simulink model "uncontrolled_test"  (R2020b)
settings: Solver=VariableStepAuto  StartTime=0.0  StopTime=5000  RelTol=1e-3
values from neighbouring files (symbols this model uses):
  spacecraft = struct()    [setup.m]
undefined symbols (not defined in the file or in its folder): constants
libraries: library x5, vrlib x3
settings Model: Creator=loren  LastModifiedBy=loren

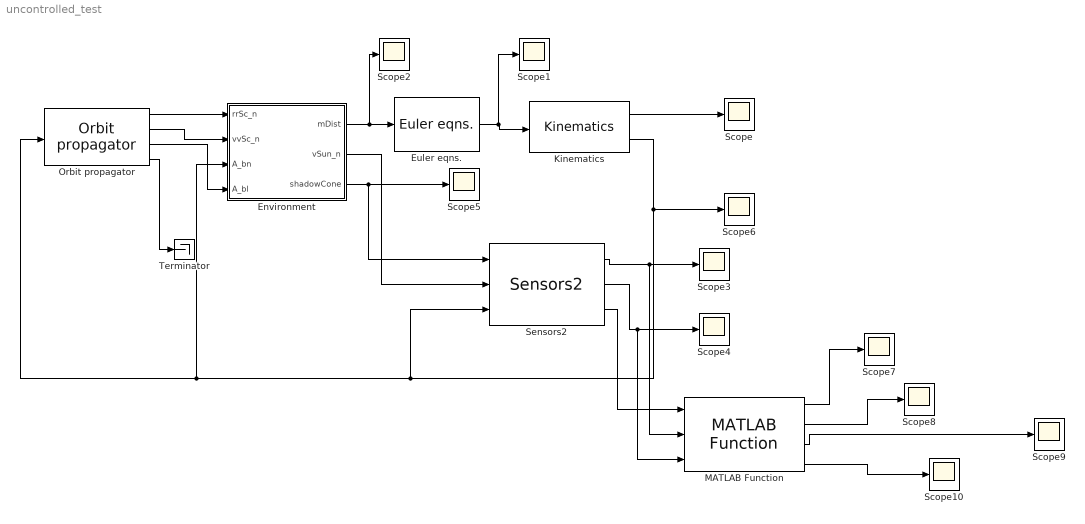
== system uncontrolled_test ==
  Environment : Subsystem  AncestorBlock=library/Environment
  Euler eqns. : library/Euler eqns.  SystemSampleTime=-1  VariantActivationTime=update diagram  Latency=0  AutoFrameSizeCalculation=off
  Kinematics : library/Kinematics  SystemSampleTime=-1  VariantActivationTime=update diagram  Latency=0  AutoFrameSizeCalculation=off
  MATLAB Function : library/MATLAB Function  SystemSampleTime=-1  VariantActivationTime=update diagram  Latency=0  AutoFrameSizeCalculation=off
      settings: SourceProductBaseCode=SL
  Orbit propagator : library/Orbit propagator  SystemSampleTime=-1  VariantActivationTime=update diagram  Latency=0  AutoFrameSizeCalculation=off
  Scope{,1..10} (11 alike) : Scope
  Sensors2 : library/Sensors2  SystemSampleTime=-1  VariantActivationTime=update diagram  Latency=0  AutoFrameSizeCalculation=off
  Terminator : Terminator
  wires:
  Orbit propagator/1 -> Environment/1(rrSc_n)
  Orbit propagator/2 -> Environment/2(vvSc_n)
  Orbit propagator/3 -> Environment/4(A_bl)
  Environment/3(shadowCone) -> Sensors2/1, Scope5/1
  Environment/1(mDist) -> Scope2/1, Euler eqns./1
  Euler eqns./1 -> Scope1/1, Kinematics/1
  Kinematics/2 -> Scope6/1, Sensors2/3, Environment/3(A_bn), Orbit propagator/1
  Environment/2(vSun_n) -> Sensors2/2
  Kinematics/1 -> Scope/1
  Orbit propagator/4 -> Terminator/1
  Sensors2/1 -> MATLAB Function/2, Scope3/1
  Sensors2/2 -> MATLAB Function/3, Scope4/1
  Sensors2/3 -> MATLAB Function/1
  MATLAB Function/1 -> Scope7/1
  MATLAB Function/2 -> Scope8/1
  MATLAB Function/3 -> Scope9/1
  MATLAB Function/4 -> Scope10/1

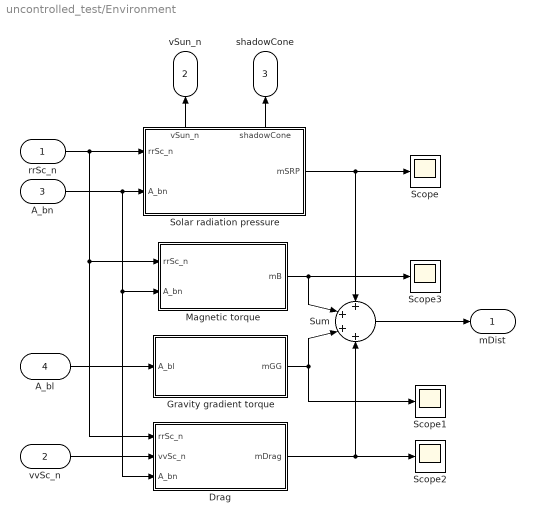
== system uncontrolled_test/Environment ==
  rrSc_n : Inport
  vvSc_n : Inport  Port=2
  A_bn : Inport  Port=3
  A_bl : Inport  Port=4
  Drag : Subsystem
  Gravity gradient torque : Subsystem
  Magnetic torque : Subsystem
  Scope{,1..3} (4 alike) : Scope
  Solar radiation pressure : Subsystem
      settings: PortSchema="{\"entries\":[{\"content\":{\"sides\":[{\"content\":{\"connectorIds\":[\"In1\",\"In2\"]},\"type\":\"ConnectorPlacement.EquallySpacedRectSide\",\"uuid\":\"1c58e148-737e-4c26-8467-bf4a1427bac3\"},{\"content\":{\"connectorIds\":[\"Out1\"],\"side\":\"RIGHT\"},\"type\":\"ConnectorPlacement.EquallySpacedRectSide\",\"uuid\":\"1132a1c1-392d-4550-8b40-4ae647f3a6c1\"},{\"content\":{\"connectorIds\":[\"Out2\",\"Out3\"],\"side\":\"TOP\"},\"type\":\"ConnectorPlacement.EquallySpacedRectSide\",\"uuid\":\"8cec875a-7b2b-408d-843f-f50e353248f2\"},{\"content\":{\"connectorIds\":[],\"side\":\"HIDDEN\"},\"type\":\"ConnectorPlacement.EquallySpacedRectSide\",\"uuid\":\"95559ba3-4215-4144-a5e7-008848b1ca72\"}]},\"type\":\"ConnectorPlacement.EquallySpacedConnector\",\"uuid\":\"cb15f690-b6d7-424c-84c7-df23a46a4e4f\"}],\"packageUris\":[\"http://schema.mathworks.com/mf0/Connector/R2020b\"],\"version\":\"1.0\"}"
  Sum : Sum  Inputs=++++
  mDist : Outport
  vSun_n : Outport  Port=2
  shadowCone : Outport  Port=3
  wires:
  Solar radiation pressure/3(shadowCone) -> shadowCone/1
  Solar radiation pressure/2(vSun_n) -> vSun_n/1
  A_bl/1 -> Gravity gradient torque/1(A_bl)
  Sum/1 -> mDist/1
  Magnetic torque/1(mB) -> Sum/2, Scope3/1
  Drag/1(mDrag) -> Sum/4, Scope2/1
  Gravity gradient torque/1(mGG) -> Sum/3, Scope1/1
  rrSc_n/1 -> Solar radiation pressure/1(rrSc_n), Magnetic torque/1(rrSc_n), Drag/1(rrSc_n)
  vvSc_n/1 -> Drag/2(vvSc_n)
  A_bn/1 -> Solar radiation pressure/2(A_bn), Magnetic torque/2(A_bn), Drag/3(A_bn)
  Solar radiation pressure/1(mSRP) -> Sum/1, Scope/1

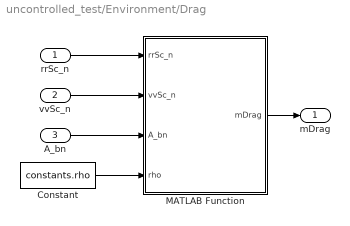
== system uncontrolled_test/Environment/Drag ==
  rrSc_n : Inport
  vvSc_n : Inport  Port=2
  A_bn : Inport  Port=3
  Constant : Constant  Value=constants.rho
  MATLAB Function : MATLAB Function  TreatAsAtomicUnit=on
  mDrag : Outport
  wires:
  Constant/1 -> MATLAB Function/4(rho)
  A_bn/1 -> MATLAB Function/3(A_bn)
  vvSc_n/1 -> MATLAB Function/2(vvSc_n)
  MATLAB Function/1(mDrag) -> mDrag/1
  rrSc_n/1 -> MATLAB Function/1(rrSc_n)

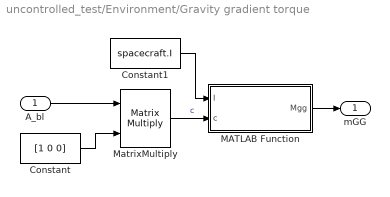
== system uncontrolled_test/Environment/Gravity gradient torque ==
  A_bl : Inport
  Constant : Constant  Value=[1 0 0]
  Constant1 : Constant  Value=spacecraft.I
  MATLAB Function : MATLAB Function  TreatAsAtomicUnit=on
  MatrixMultiply : Product  Multiplication=Matrix(*)
  mGG : Outport
  wires:
  A_bl/1 -> MatrixMultiply/1
  MATLAB Function/1(Mgg) -> mGG/1
  MatrixMultiply/1 -> MATLAB Function/2(c)  "c"
  Constant/1 -> MatrixMultiply/2
  Constant1/1 -> MATLAB Function/1(I)

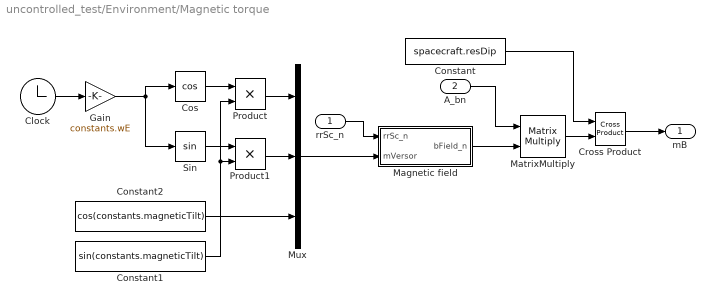
== system uncontrolled_test/Environment/Magnetic torque ==
  rrSc_n : Inport
  A_bn : Inport  Port=2
  Clock : Clock
  Constant : Constant  Value=spacecraft.resDip
  Constant1 : Constant  Value=sin(constants.magneticTilt)
  Constant2 : Constant  Value=cos(constants.magneticTilt)
  Cos : Trigonometry  Operator=cos
  Cross Product : vrlib/Utilities/Cross Product
  Gain : Gain  Gain=constants.wE
  Magnetic field : Subsystem
  MatrixMultiply : Product  Multiplication=Matrix(*)
  Mux : Mux  Inputs=3
  Product : Product
  Product1 : Product
  Sin : Trigonometry
  mB : Outport
  wires:
  Cross Product/1 -> mB/1
  MatrixMultiply/1 -> Cross Product/2
  Magnetic field/1(bField_n) -> MatrixMultiply/2
  Mux/1 -> Magnetic field/2(mVersor)
  rrSc_n/1 -> Magnetic field/1(rrSc_n)
  A_bn/1 -> MatrixMultiply/1
  Constant1/1 -> Product1/2, Product/2
  Product1/1 -> Mux/2
  Product/1 -> Mux/1
  Cos/1 -> Product/1
  Sin/1 -> Product1/1
  Constant2/1 -> Mux/3
  Gain/1 -> Cos/1, Sin/1
  Constant/1 -> Cross Product/1
  Clock/1 -> Gain/1

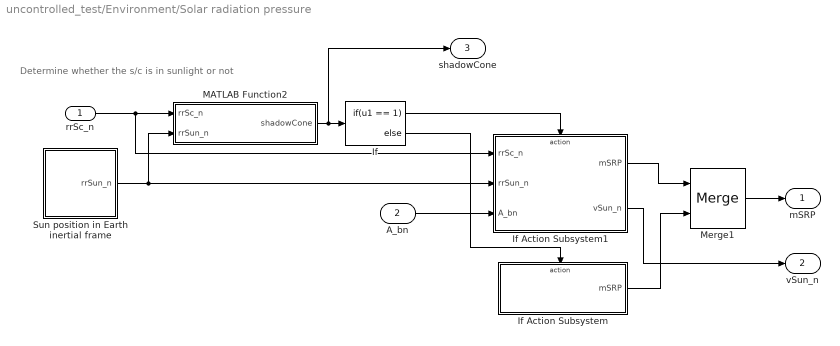
== system uncontrolled_test/Environment/Solar radiation pressure ==
  note: Determine whether the s/c is in sunlight or not
  rrSc_n : Inport
  A_bn : Inport  Port=2
  If : If  IfExpression=u1 == 1
  If Action Subsystem : Subsystem  TreatAsAtomicUnit=on
  If Action Subsystem1 : Subsystem  TreatAsAtomicUnit=on
  MATLAB Function2 : MATLAB Function  TreatAsAtomicUnit=on
  Merge1 : Merge
  Sun position in Earth inertial frame : Subsystem
  mSRP : Outport
  vSun_n : Outport  Port=2
  shadowCone : Outport  Port=3
  wires:
  If Action Subsystem1/2(vSun_n) -> vSun_n/1
  Sun position in Earth inertial frame/1(rrSun_n) -> MATLAB Function2/2(rrSun_n), If Action Subsystem1/2(rrSun_n)
  A_bn/1 -> If Action Subsystem1/3(A_bn)
  If Action Subsystem1/1(mSRP) -> Merge1/1
  Merge1/1 -> mSRP/1
  rrSc_n/1 -> MATLAB Function2/1(rrSc_n), If Action Subsystem1/1(rrSc_n)
  If Action Subsystem/1(mSRP) -> Merge1/2
  If/1 -> If Action Subsystem1/Action
  If/2 -> If Action Subsystem/Action
  MATLAB Function2/1(shadowCone) -> If/1, shadowCone/1

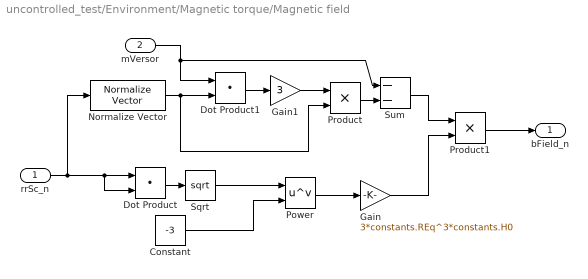
== system uncontrolled_test/Environment/Magnetic torque/Magnetic field ==
  rrSc_n : Inport
  mVersor : Inport  Port=2
  Constant : Constant  Value=-3
  Dot Product : DotProduct  InputSameDT=on  OutDataTypeStr=Inherit: Inherit via internal rule
  Dot Product1 : DotProduct  InputSameDT=on  OutDataTypeStr=Inherit: Inherit via internal rule
  Gain : Gain  Gain=3*constants.REq^3*constants.H0
  Gain1 : Gain  Gain=3
  Normalize Vector : vrlib/Utilities/Normalize Vector  maxzero=0
  Power : Math  Operator=pow  SaturateOnIntegerOverflow=on
  Product : Product
  Product1 : Product
  Sqrt : Sqrt  SaturateOnIntegerOverflow=on
  Sum : Sum  Inputs=--
  bField_n : Outport
  wires:
  Product1/1 -> bField_n/1
  Gain/1 -> Product1/2
  Sum/1 -> Product1/1
  Product/1 -> Sum/2
  Gain1/1 -> Product/1
  Dot Product1/1 -> Gain1/1
  mVersor/1 -> Dot Product1/1, Sum/1
  Normalize Vector/1 -> Dot Product1/2, Product/2
  Power/1 -> Gain/1
  Sqrt/1 -> Power/1
  Dot Product/1 -> Sqrt/1
  Constant/1 -> Power/2
  rrSc_n/1 -> Dot Product/1, Dot Product/2, Normalize Vector/1

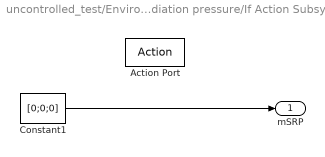
== system uncontrolled_test/Environment/Solar radiation pressure/If Action Subsystem ==
  Action Port : ActionPort  ActionPortLabel=else
  Constant1 : Constant  Value=[0;0;0]
  mSRP : Outport
  wires:
  Constant1/1 -> mSRP/1

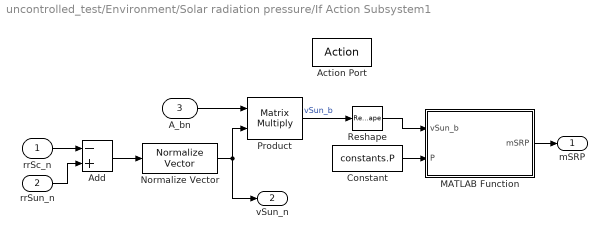
== system uncontrolled_test/Environment/Solar radiation pressure/If Action Subsystem1 ==
  rrSc_n : Inport
  rrSun_n : Inport  Port=2
  A_bn : Inport  Port=3
  Action Port : ActionPort  ActionPortLabel=if(u1 == 1)
  Add : Sum  Inputs=-+
  Constant : Constant  Value=constants.P
  MATLAB Function : MATLAB Function  TreatAsAtomicUnit=on
  Normalize Vector : vrlib/Utilities/Normalize Vector  maxzero=0
  Product : Product  Multiplication=Matrix(*)
  Reshape : Reshape  OutputDimensionality=Column vector (2-D)
  mSRP : Outport
  vSun_n : Outport  Port=2
  wires:
  Reshape/1 -> MATLAB Function/1(vSun_b)
  Constant/1 -> MATLAB Function/2(P)
  rrSc_n/1 -> Add/1
  MATLAB Function/1(mSRP) -> mSRP/1
  Add/1 -> Normalize Vector/1
  Normalize Vector/1 -> Product/2, vSun_n/1
  Product/1 -> Reshape/1  "vSun_b"
  rrSun_n/1 -> Add/2
  A_bn/1 -> Product/1

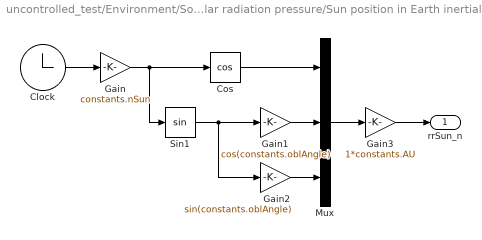
== system uncontrolled_test/Environment/Solar radiation pressure/Sun position in Earth inertial frame ==
  Clock : Clock
  Cos : Trigonometry  Operator=cos
  Gain : Gain  Gain=constants.nSun
  Gain1 : Gain  Gain=cos(constants.oblAngle)
  Gain2 : Gain  Gain=sin(constants.oblAngle)
  Gain3 : Gain  Gain=1*constants.AU
  Mux : Mux  Inputs=3
  Sin1 : Trigonometry
  rrSun_n : Outport
  wires:
  Gain3/1 -> rrSun_n/1
  Cos/1 -> Mux/1
  Sin1/1 -> Gain1/1, Gain2/1
  Mux/1 -> Gain3/1
  Gain1/1 -> Mux/2
  Gain/1 -> Cos/1, Sin1/1
  Clock/1 -> Gain/1
  Gain2/1 -> Mux/3

== matlab function uncontrolled_test/Environment/Gravity gradient torque/MATLAB Function ==
  data: Mgg output; I input; c input
function Mgg = gravity_gradient(I, c)

mu = 398600;
REq = 6371.8e3;

c1 = c(1);
c2 = c(2);
c3 = c(3);
Ix = I(1,1);
Iy = I(2,2);
Iz = I(3,3);

Mgg = 3*mu/(REq^3)*[(Iz - Iy)*c2*c3;...
    (Ix - Iz)*c1*c3;...
    (Iy - Ix)*c1*c2];

end

== matlab function uncontrolled_test/Environment/Solar radiation pressure/If Action Subsystem1/MATLAB Function ==
  data: vSun_b input; P input; mSRP output; surfaces parameter
function mSRP = srp(vSun_b, P, surfaces)

rSurf = surfaces.rSurf;
n = surfaces.n;
A = surfaces.A;
rhoS = surfaces.rhoS;
rhoD = surfaces.rhoD;

mSRP = zeros(3,1);

for k = 1:size(rSurf,1)
    n_b = n(:,k);
    s_dot = dot(vSun_b, n_b);
    if s_dot > 0
        rhoS_temp = rhoS(k);
        Fsrp_i = - P*A(k)*s_dot.*((1-rhoS_temp).*vSun_b +...
            (2*rhoS_temp*s_dot + 2/3*rhoD(k)).*n_b);
        mSRP = mSRP + cross(rSurf(:,k), Fsrp_i);
    end
end

% aggiungere questione su "ombra"

end

== matlab function uncontrolled_test/Environment/Drag/MATLAB Function ==
  data: rrSc_n input; mDrag output; vvSc_n input; A_bn input; rho input; surfaces parameter
function  mDrag = drag(rrSc_n, vvSc_n, A_bn, rho, surfaces)

rSurf = surfaces.rSurf;
n = surfaces.n;
A = surfaces.A;
cd = surfaces.cd;

wE = 7.2921150e-5; %[rad/s]
vvRel_n = [vvSc_n(1) + wE*rrSc_n(2); vvSc_n(2) - wE*rrSc_n(1); vvSc_n(3)];
vvRel_b = A_bn*vvRel_n;

vRel = norm(vvRel_n);
vRel_b = norm(vvRel_b);
vvVersor = vvRel_b/vRel_b;

c = -1/2*rho*cd*vRel^2.*vvVersor;

mDrag = zeros(3,1);

for k = 1:size(rSurf,1)
        n_dot = dot(n(:,k), vvVersor);
    if n_dot > 0
        A_cross = A(k)*n_dot;
        Fdrag_i = c*A_cross;
        mDrag = mDrag + cross(rSurf(:,k), Fdrag_i);
    end
end

end

== matlab function uncontrolled_test/Environment/Solar radiation pressure/MATLAB Function2 ==
  data: rrSc_n input; shadowCone output; rrSun_n input
function shadowCone = cone(rrSc_n, rrSun_n)

% PROTOTYPE:
%  shadow_cone = cone(rr_sc, rr_sun_n)
% 
% DESCRIPTION:
%   This function returns a parameter that is 1 if the s/c is out of the 
%   planet's shadow cone (SRP effects considerable) or 0 if the s/c is 
%   inside the planet's shadow cone (NO SRP)
% 
% INPUT:
% rr_sc:            geocentric position vector of the s/c
% rr_sun_n:        geocentric position vector of the sun
%
% OUTPUT:
% shadow_cone:      boolean parameter (0 or 1)
%
% CONTRIBUTORS:
% Velo Giacomo
%
% VERSIONS:
% 2019-12-10 first version
%
% CALLED FUNCTIONS:
%     none


Req = 6378.1;
r = norm(rrSc_n);     
r_sun = norm(rrSun_n);
% Angle between s/c geocentric position and the tangent to Earth's surface
theta_sc = acos(Req/r);
% Angle between sun geocentric position and the tangent to Earth's surface
theta_sun = acos(Req/r_sun);
% Angle between s/c geocentric position and sun geocentric position
theta = acos(dot(rrSc_n, rrSun_n)/(r*r_sun));

% If the s/c is inside the shadow cone of the planet the value of
% shadow_cone will be = 0

    if theta_sc + theta_sun <= theta
        shadowCone = 0;
    else
        shadowCone = 1;
    end

end
